simulink model "wireless_chain_sol"  (R2023b)
settings: Solver=FixedStepAuto  StartTime=0.0  StopTime=Inf  FixedStep=sample_time  RelTol=1e-3
InitFcn:
  | init_fcn
StopFcn:
  | stop_fcn
undefined symbols (not defined in the file): entity, getAttribute, m, timeStamp
libraries: simulink x1, dspstat3 x1, dspsigops x1
settings Model: Creator=jorge  LastModifiedBy=jorge
settings OptimizationCC: ReuseModelBlockBuffer=off

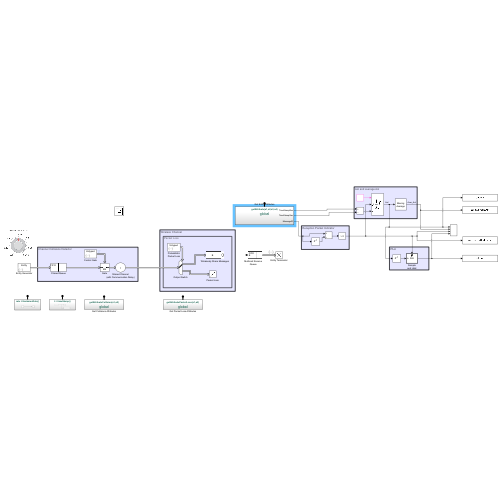
[thumbnail: Simulink's stored preview of the top-level diagram]
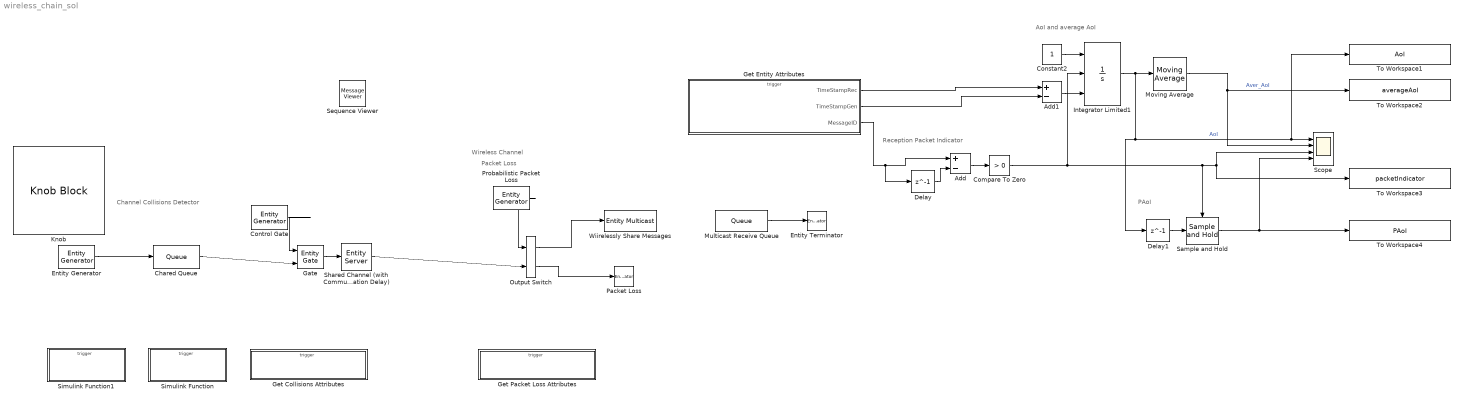
== system wireless_chain_sol ==
  note: Reception Packet Indicator
  note: AoI and average AoI
  note: PAoI
  note: Wireless Channel
  note: Channel Collisions Detector
  note: Packet Loss
  Add : Sum  Inputs=+-
  Add1 : Sum  Inputs=+-
  Chared Queue : Queue  InputPortMessageModes=m  OutputPortMessageModes=m  Capacity=Inf
  Compare To Zero : simulink/Logic and Bit Operations/Compare To Zero  relop=>  OutDataTypeStr=boolean
  Constant2 : Constant
  Control Gate : EntityGenerator  OutputPortMessageModes=m  TimeSource=MATLAB action  Period=0.2  IntergenerationTimeAction=|  GenerateAction=|  AttributeName=entity  EntityTypeName=EntityGate  DataInitialValue=1
      IntergenerationTimeAction=|
      | % Current channel failure state 
      | % (true - failed, false - operational)
      | persistent failure; 
      | if isempty(failure)
      |     % Initial condition: channel is operational.
      |     failure = false;
      | end
      | 
      | if failure
      |     % Repair time is an uniformly distributed random
      |     % variable between 1 and 2.
      |     dt = randi([1 2],1,1);
      | else
      |     % Duration between failures is a uniformly
      |     % distributed random variable between 1 and 10.
      |     dt = randi([1 10],1,1);
      | end
      | 
      | % Update failure state.
      | failure = ~failure;
      GenerateAction=|
      | persistent gateControl;
      | if isempty(gateControl)
      |     gateControl = 1;
      | end
      | entity = gateControl;
      | gateControl = 1-gateControl;
      | 
      | %stamping each generated packet with the clock
      | getAttributeCollision(entity,timeStamp());
  Delay : Delay  DelayLength=1
  Delay1 : Delay  DelayLength=1
  Entity Generator : EntityGenerator  OutputPortMessageModes=m  TimeSource=MATLAB action  IntergenerationTimeAction=|  GenerateAction=|  AttributeName=Data|TimeStampGeneration|TimeStampServiceComplete|TotalTime|MessageID  AttributeInitialValue=uint8(zeros(1,length(message)))|0|0|0|0  EntityType=Structured  EntityTypeName=Entity
      IntergenerationTimeAction=|
      | % dt = rand(1,1);
      | %dt = randi([0 10],1,1);
      | %dt=5;
      | dt=1/EmissionRate();
      GenerateAction=|
      | %stamping each generated packet with the clock
      | entity.TimeStampGeneration = timeStamp();
      | %stamping each generated packet with an ID
      | persistent counter;
      | 
      | if isempty(counter)
      |     counter=1;
      | end
      | 
      | entity.MessageID=counter;
      | counter=counter+1;
  Entity Terminator : EntityTerminator  InputPortMessageModes=m  EntryAction=getAttribute(entity.Data',entity.MessageID,entity.TimeStampGeneration,timeStamp());
  Gate : EntityGate  InputPortMessageModes=m,m  OutputPortMessageModes=m  OpenGateAtSimulationStart=on
  Get Collisions Attributes : Subsystem  TreatAsAtomicUnit=on
  Get Entity Attributes : Subsystem  TreatAsAtomicUnit=on
  Get Packet Loss Attributes : Subsystem  TreatAsAtomicUnit=on
  Integrator Limited1 : Integrator  ExternalReset=rising  InitialConditionSource=external  LimitOutput=on  UpperSaturationLimit=1000  LowerSaturationLimit=0
  Knob : KnobBlock  ScaleMin=0.10000000000000001  ScaleMax=0.999
  Moving Average : dspstat3/Moving Average  Method=Sliding window  ForgettingFactorPort=off  SpecifyWindowLength=on  WindowLength=50000  OverlapLength=49999  AllowArbitraryInputLength=off  ForgettingFactor=0.9  SimulateUsing=Code generation
  Multicast Receive Queue : Queue  OutputPortMessageModes=m  EntityArrivalSource=Multicast  MulticastTag=B
  Output Switch : EntityOutputSwitch  InputPortMessageModes=m,m  OutputPortMessageModes=m,m  SwitchingCriterion=From control port  SwitchAttributeName=Attribute1
      settings: InputPortMap=u0,u1
  Packet Loss : EntityTerminator  InputPortMessageModes=m
  Probabilistic Packet Loss : EntityGenerator  OutputPortMessageModes=m  GenerateAction=|  AttributeName=entity  EntityTypeName=Entity  DataInitialValue=1
      | persistent rngInit;
      |    if isempty(rngInit)
      |        seed = 12345;
      |        rng(seed);
      |        rngInit = true;
      |    end
      | 
      |    % Pattern: Uniform distribution
      |    % m: Minimum, M: Maximum
      |    m = 0; M = 1;
      |    x = m + (M - m) * rand;
      |    % x is generated from uniform distribution and 
      |    % takes values between |0| and |1|.
      |    if x > 0.1  
      |       % Entity carries data |1| and this forces Output switch to select 
      |       % output |1| that forwards a message to a receive component.
      |       entity  = 1;  
      |    else
      |       % Entity carries data |2| and this forces Output switch to select 
      |       % output |2| and this represents a packet loss.
      |       entity = 2;    
      |       %stamping each generated packet with the clock
      |       getAttributePacketLoss(entity,timeStamp());
      |    end
  Sample and Hold : dspsigops/Sample and Hold  trig=Rising edge  initCond=0  latchinput=off
  Scope : Scope  NumInputPorts=4
  Sequence Viewer : MessageViewer  History=1000  SavedRootId=#
  Shared Channel (with Communication Delay) : EntityServer  InputPortMessageModes=m  OutputPortMessageModes=m  Capacity=1  ServiceTimeValue=1
  Simulink Function : Subsystem  TreatAsAtomicUnit=on
  Simulink Function1 : Subsystem  TreatAsAtomicUnit=on
  To Workspace1 : ToWorkspace  VariableName=AoI  SaveFormat=Timeseries  SampleTime=-1
  To Workspace2 : ToWorkspace  VariableName=averageAoI  SaveFormat=Timeseries  SampleTime=-1
  To Workspace3 : ToWorkspace  VariableName=packetIndicator  SaveFormat=Timeseries  SampleTime=-1
  To Workspace4 : ToWorkspace  VariableName=PAoI  SaveFormat=Timeseries  SampleTime=-1
  Wiirelessly Share Messages : EntityMulticast  InputPortMessageModes=m  MulticastTag=B
  wires:
  Multicast Receive Queue/1 -> Entity Terminator/1
  Output Switch/1 -> Wiirelessly Share Messages/1
  Chared Queue/1 -> Gate/2
  Output Switch/2 -> Packet Loss/1
  Shared Channel (with Communication Delay)/1 -> Output Switch/2
  Probabilistic Packet Loss/1 -> Output Switch/1
  Gate/1 -> Shared Channel (with Communication Delay)/1
  Control Gate/1 -> Gate/1
  Entity Generator/1 -> Chared Queue/1
  Sample and Hold/1 -> To Workspace4/1, Scope/4
  Delay1/1 -> Sample and Hold/1
  Get Entity Attributes/1(TimeStampRec) -> Add1/1
  Add1/1 -> Integrator Limited1/3
  Moving Average/1 -> To Workspace2/1, Scope/2  "Aver_AoI"
  Get Entity Attributes/2(TimeStampGen) -> Add1/2
  Constant2/1 -> Integrator Limited1/1
  Integrator Limited1/1 -> Delay1/1, To Workspace1/1, Scope/1, Moving Average/1  "AoI"
  Compare To Zero/1 -> Sample and Hold/Trigger, To Workspace3/1, Scope/3, Integrator Limited1/2
  Delay/1 -> Add/2
  Add/1 -> Compare To Zero/1
  Get Entity Attributes/3(MessageID) -> Delay/1, Add/1

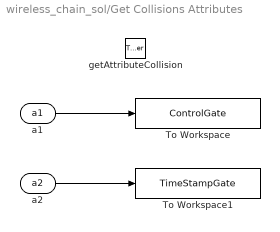
== system wireless_chain_sol/Get Collisions Attributes ==
  getAttributeCollision : TriggerPort  TriggerType=function-call  IsSimulinkFunction=on  FunctionName=getAttributeCollision  VariantControl=Variant
  To Workspace : ToWorkspace  VariableName=ControlGate  SaveFormat=Timeseries  SampleTime=-1
  To Workspace1 : ToWorkspace  VariableName=TimeStampGate  SaveFormat=Timeseries  SampleTime=-1
  a1 : ArgIn  ArgumentName=a1
  a2 : ArgIn  Port=2  ArgumentName=a2
  wires:
  a1/1 -> To Workspace/1
  a2/1 -> To Workspace1/1

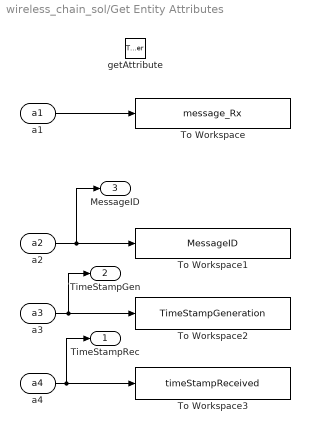
== system wireless_chain_sol/Get Entity Attributes ==
  getAttribute : TriggerPort  TriggerType=function-call  IsSimulinkFunction=on  FunctionName=getAttribute  VariantControl=Variant
  To Workspace : ToWorkspace  VariableName=message_Rx  SaveFormat=Timeseries  SampleTime=-1
  To Workspace1 : ToWorkspace  VariableName=MessageID  SaveFormat=Timeseries  SampleTime=-1
  To Workspace2 : ToWorkspace  VariableName=TimeStampGeneration  SaveFormat=Timeseries  SampleTime=-1
  To Workspace3 : ToWorkspace  VariableName=timeStampReceived  SaveFormat=Timeseries  SampleTime=-1
  a1 : ArgIn  OutDataTypeStr=uint8  PortDimensions=12  ArgumentName=a1
  a2 : ArgIn  Port=2  ArgumentName=a2
  a3 : ArgIn  Port=3  ArgumentName=a3
  a4 : ArgIn  Port=4  ArgumentName=a4
  TimeStampRec : Outport
  TimeStampGen : Outport  Port=2
  MessageID : Outport  Port=3
  wires:
  a1/1 -> To Workspace/1
  a3/1 -> TimeStampGen/1, To Workspace2/1
  a4/1 -> TimeStampRec/1, To Workspace3/1
  a2/1 -> MessageID/1, To Workspace1/1

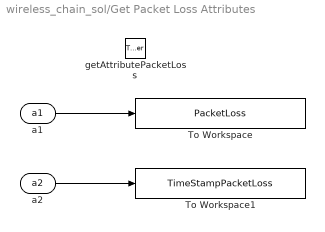
== system wireless_chain_sol/Get Packet Loss Attributes ==
  getAttributePacketLoss : TriggerPort  TriggerType=function-call  IsSimulinkFunction=on  FunctionName=getAttributePacketLoss  VariantControl=Variant
  To Workspace : ToWorkspace  VariableName=PacketLoss  SaveFormat=Timeseries  SampleTime=-1
  To Workspace1 : ToWorkspace  VariableName=TimeStampPacketLoss  SaveFormat=Timeseries  SampleTime=-1
  a1 : ArgIn  ArgumentName=a1
  a2 : ArgIn  Port=2  ArgumentName=a2
  wires:
  a1/1 -> To Workspace/1
  a2/1 -> To Workspace1/1

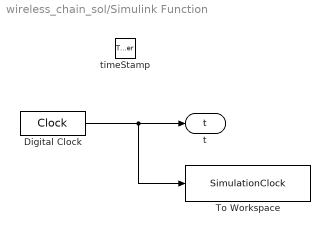
== system wireless_chain_sol/Simulink Function ==
  timeStamp : TriggerPort  TriggerType=function-call  IsSimulinkFunction=on  FunctionName=timeStamp  FunctionVisibility=scoped  VariantControl=(inherit)
  Digital Clock : DigitalClock  SampleTime=-1
  To Workspace : ToWorkspace  VariableName=SimulationClock  SaveFormat=Timeseries  SampleTime=-1
  t : ArgOut  DisableCoverage=on  ArgumentName=t
  wires:
  Digital Clock/1 -> To Workspace/1, t/1

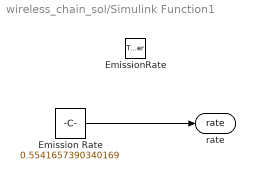
== system wireless_chain_sol/Simulink Function1 ==
  EmissionRate : TriggerPort  TriggerType=function-call  IsSimulinkFunction=on  FunctionName=EmissionRate  FunctionVisibility=scoped  VariantControl=(inherit)
  Emission Rate : Constant  Value=0.5541657390340169
  rate : ArgOut  DisableCoverage=on  ArgumentName=rate
  wires:
  Emission Rate/1 -> rate/1
